simulink model "ftm_incremental_encoder_s32k1xx"  (Simulink 9.0)
settings: Solver=FixedStepDiscrete  StartTime=0.0  StopTime=10.0  FixedStep=0.01  RelTol=1e-3  EnableMultiTasking=on
model workspace (MAT data in the model file):
  FTM_Max_Counter = 4096
  Number_of_Divisions = 1024
  Sampling_Time = 0.01
  Scale_Factor : num (value not decoded)
InitFcn:
  | mbd_s32k_consistency_checks(bdroot(gcs));
undefined symbols (not defined in the file): LQFP
libraries: mbd_s32k1xx_ec_toolbox x7, simulink x1
Description:
  | This model shows FlexTimer's Quadrature Decoder Mode.
  | 
  | The Quadrature Encoder signals of a running motor are emulated using the
  | block called "Signal_Generation" using the FTM PWM. The FTM PWM writes
  | the output on the pins PTD15, and PTD0.
  | 
  | The FTM Quadrature Decoder block has as input the pins PTA1, and PTB2.
  | 
  | For the example to work connect PTA1 to PTD15 and PTB2 to PTD0.
  | 
  | This example has also a FreeMaster project associated, which is called
  | "ftm_incremental_encoder_s32k1xx.pmp".
  | 
  | For a given value of "Speed_Command" variable the pins PTD15, and PTD0
  | will be the same values as the signals of Quadrature Encoder of a
  | spinning motor at the speed "Speed_Command". It's value can be modified
  | from FreeMaster.
  | 
  | Validation: In FreeMaster "Motor_Speed" should be equal to "Speed_Command".
settings Model: Creator=NXP MBDT Team  LastModifiedBy=nxf35172  OrderedModelArguments=off
settings DataIOCC: ExternalInput=off  InitialState=off  LimitDataPoints=on  SaveOutput=off  SignalLogging=off  SaveTime=off
settings OptimizationCC: DefaultParameterBehavior=Inlined  LifeSpan=1
settings DebuggingCC: SolverPrmCheckMsg=warning  InheritedTsInSrcMsg=none  SingleTaskRateTransMsg=error  UnconnectedInputMsg=error  UnconnectedOutputMsg=error  UnconnectedLineMsg=error  AllowSymbolicDim=off  UnknownTsInhSupMsg=error  StateNameClashWarn=warning
settings HardwareCC: ProdLargestAtomicInteger=Long  ProdLargestAtomicFloat=Double  ProdEndianess=LittleEndian  ProdHWDeviceType=ARM Compatible->ARM Cortex
settings SFSimCC: MATLABDynamicMemAlloc=off
settings RTWCC: SystemTargetFile=mbd_s32k.tlc  MakeCommand=mbd_s32k_make_rtw COPY_MDLREF_INCLUDES=0  TemplateMakefile=mbd_s32k.tmf  Description=Model Based Design Toolbox S32K14x Code Generation Target  GenerateReport=on  LaunchReport=on
settings CodeAppCC: IgnoreCustomStorageClasses=off
settings STFCustomTargetCC: CombineOutputUpdateFcns=on  ERTCustomFileBanners=on  SupportContinuousTime=off  SupportNonInlinedSFcns=off  RemoveResetFunc=on  MATLABClassNameForMDSCustomization=Simulink.SoftwareTarget.ERTCustomization  GRTInterface=off  SystemTargetFile=mbd_s32k14.tlc
settings ERTTargetCC: MultiwordLength=2048  ParMdlRefBuildCompliant=off  CompOptLevelCompliant=off  ConcurrentExecutionCompliant=off  ModelStepFunctionPrototypeControlCompliant=off  CPPClassGenCompliant=off  UseToolchainInfoCompliant=off  InlinedParameterPlacement=NonHierarchical  ERTCustomFileTemplate=example_file_process.tlc  ConvertIfToSwitch=off  SuppressUnreachableDefaultCases=off

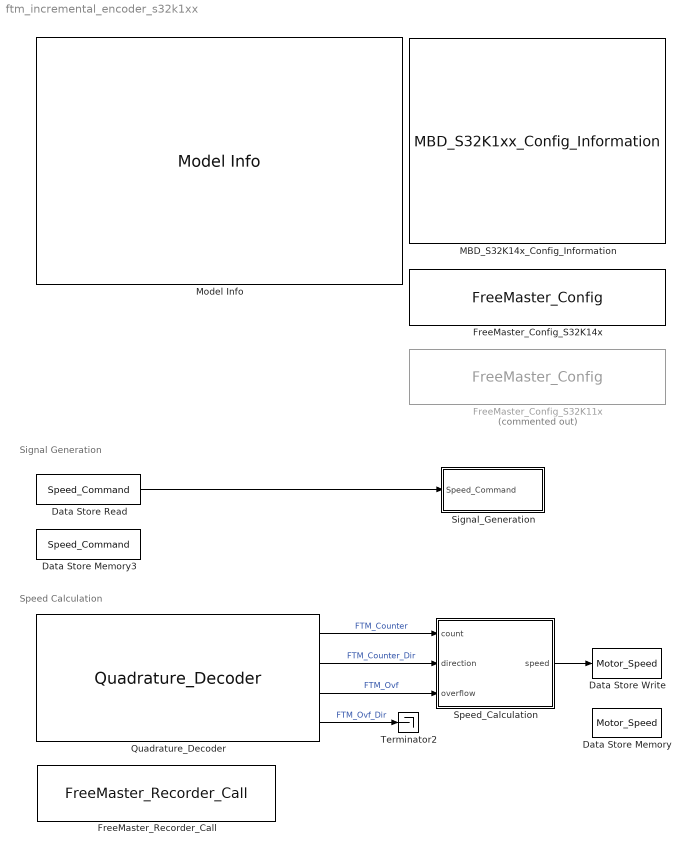
== system ftm_incremental_encoder_s32k1xx ==
  note: Signal Generation
  note: Speed Calculation
  Data Store Memory : DataStoreMemory  DataStoreName=Motor_Speed  ReadBeforeWriteMsg=warning  WriteAfterWriteMsg=warning  WriteAfterReadMsg=warning  ShowAdditionalParam=off
  Data Store Memory3 : DataStoreMemory  DataStoreName=Speed_Command  ReadBeforeWriteMsg=warning  WriteAfterWriteMsg=warning  WriteAfterReadMsg=warning  InitialValue=500  ShowAdditionalParam=off  OutDataTypeStr=single
  Data Store Read : DataStoreRead  DataStoreName=Speed_Command
  Data Store Write : DataStoreWrite  DataStoreName=Motor_Speed  DataStoreElements=Motor_Speed
  FreeMaster_Config_S32K11x : mbd_s32k1xx_ec_toolbox/Utility Blocks/FreeMaster_Config  Commented=on  interface=LPUART0  baudrate=57600  rxd=PTB0: [LPUART0_RX | Receive]  txd=PTB1: [LPUART0_TX | Transmit]  mode=Short Interrupt  isr_prio=1  show_adv_opts=on  use_scope=on  max_scope_vars=8  use_recorder=on  max_rec_vars=8  rec_buff_size=1024  rec_timebase=0 milliseconds  comm_buffer_size_auto=on  comm_buffer_size=255  comm_rqueue_size_default=on  comm_rqueue_size=32
  FreeMaster_Config_S32K14x : mbd_s32k1xx_ec_toolbox/Utility Blocks/FreeMaster_Config  interface=LPUART1  baudrate=57600  rxd=PTC6: [LPUART1_RX | Receive]  txd=PTC7: [LPUART1_TX | Transmit]  mode=Short Interrupt  isr_prio=1  show_adv_opts=on  use_scope=on  max_scope_vars=8  use_recorder=on  max_rec_vars=8  rec_buff_size=1024  rec_timebase=0 milliseconds  comm_buffer_size_auto=on  comm_buffer_size=255  comm_rqueue_size_default=on  comm_rqueue_size=32
  FreeMaster_Recorder_Call : mbd_s32k1xx_ec_toolbox/Utility Blocks/FreeMaster_Recorder_Call
  MBD_S32K14x_Config_Information : mbd_s32k1xx_ec_toolbox/MBD_S32K1xx_Config_Information  mbdt_ver=0  disp_str=|  config_params=[]  mcu_target_name=S32K146  mcu_target_package=144-LQFP  mcu_target_sram_size=128KB  mcu_system_clock_freq=80  mcu_xtal_freq=External 8  mcu_steptick_timer=LPIT Channel 0  mcu_steptick_prio=0  ds_import_enable=on  target_compiler=GCC  target_memory=FLASH  gcc_target_compile_opts=-mcpu=cortex-m4 -mthumb -mfloat-abi=hard -mfpu=fpv4-sp-d16 -O1 -g -gstrict-dwarf  gcc_target_assemble_opts=-mcpu=cortex-m4 -mthumb -mfloat-abi=hard -mfpu=fpv4-sp-d16 -g  gcc_target_link_opts=-mcpu=cortex-m4 -mthumb -mfloat-abi=hard -mfpu=fpv4-sp-d16  gcc_target_default_lcf=on  gcc_target_user_lcf=S32K146_128_flash.ld  ghs_target_compile_opts=-cpu=cortexm4f -thumb -DARM_MATH_CM4 -fpu=vfpv4_d16 -fsingle -Ogeneral -Wundef -Wimplicit-int -Wshadow -Wtrigraphs --no_commons --gnu_asm -gnu99 -gdwarf-2 -G  ghs_target_assemble_opts=-cpu=cortexm4f -fpu=vfpv4_d16  ghs_target_link_opts=-cpu=cortexm4f -thumb -fpu=vfpv4_d16  ghs_target_default_lcf=off  ghs_target_user_lcf=S32K146_128_flash.ld  iar_target_compile_opts=--cpu=Cortex-M4F --thumb --fpu=VFPv4_sp -Ol -e --debug --dlib_config normal  iar_target_assemble_opts=--cpu Cortex-M4F --thumb --fpu VFPv4_sp  iar_target_link_opts=--no_exceptions --vfe --inline  iar_target_default_lcf=off  iar_target_user_lcf=S32K146_128_flash.icf  pil_download_enable=off  rbl_download_enable=on  rbl_start_delay=5000000  rbl_download_interface=OpenSDA  rbl_restart_request=off  rbl_com_port=Custom  rbl_com_port_custom=COM1  pil_download_rate=57600  pil_opensda_drive=Custom  pil_opensda_drive_custom=D  pil_uart_instance=0  pil_uart_rx=PTA2: [LPUART0_RX | Receive]  pil_uart_tx=PTA3: [LPUART0_TX | Transmit]  FTM_PWM_PcrCheckEnDis=on  FTM_Input_Edge_Inputs_PcrCheckEnDis=on  FTM_Dual_Edge_Inputs_PcrCheckEnDis=on  FTM_Quadrature_Inputs_PcrCheckEnDis=on  FTM_Hall_Sensor_Inputs_PcrCheckEnDis=on  LPTMR_PcrCheckEnDis=on  PIT_PcrCheckEnDis=on  RTC_PcrCheckEnDis=on  FlexCAN_PcrCheckEnDis=on  LIN_PcrCheckEnDis=on  FlexIO_PcrCheckEnDis=on  LPI2C_PcrCheckEnDis=on  LPSPI_PcrCheckEnDis=on  LPUART_PcrCheckEnDis=on  CMP_PcrCheckEnDis=on  GPIO_OutputPcrCheckEnDis=on  GPIO_InputPcrCheckEnDis=on  SBC_PcrCheckEnDis=on  AMMCLIB_PcrCheckEnDis=on  FM_PcrCheckEnDis=on  Profile_PcrCheckEnDis=on  ConfigParams_PcrCheckEnDis=on  ModelRef_PcrCheckEnDis=on  PDB0_PcrCheckEnDis=on  CSEc_PcrCheckEnDis=on  eDMA_PcrCheckEnDis=on  ADC_PcrCheckEnDis=on  WDOG_PcrCheckEnDis=on
      | Target : S32K144-48KB_SRAM
      | Package : 100-pin
      | System clock : 80 MHz
      | XTAL clock : External 8 MHz
      | Compiler : IAR
      | Target Type : FLASH
      | Download Code after build : off
      | Step Tick Interrupt Priority : 15
  Model Info : simulink/Model-Wide Utilities/Model Info  Frame=off  DisplayStringWithTags=|  HorizontalTextAlignment=Left  LeftAlignmentValue=0.02
      | Model Name: %<ModelName>
      | 
      | Description: %<Description>
  Quadrature_Decoder : mbd_s32k1xx_ec_toolbox/Motor Control Blocks/FTM Blocks/Quadrature_Decoder  Priority=1  ftmModule=1  ec_mode=Phase A and Phase B  prescaler=1  cntin=0  mod=4096  phA_filtr_en=off  phA_filter=0  phA_pin=PTA1: [FTM1_QD_PHA | FTM quadrature Decode PhaseA]  polA=Normal  phB_filtr_en=off  phB_filter=0  phB_pin=PTB2: [FTM1_QD_PHB | FTM quadrature Decode PhaseB]  polB=Normal
  Signal_Generation : Subsystem
  Speed_Calculation : Subsystem
  Terminator2 : Terminator
  wires:
  Quadrature_Decoder/1 -> Speed_Calculation/1(count)  "FTM_Counter"
  Quadrature_Decoder/2 -> Speed_Calculation/2(direction)  "FTM_Counter_Dir"
  Quadrature_Decoder/3 -> Speed_Calculation/3(overflow)  "FTM_Ovf"
  Quadrature_Decoder/4 -> Terminator2/1  "FTM_Ovf_Dir"
  Speed_Calculation/1(speed) -> Data Store Write/1
  Data Store Read/1 -> Signal_Generation/1(Speed_Command)

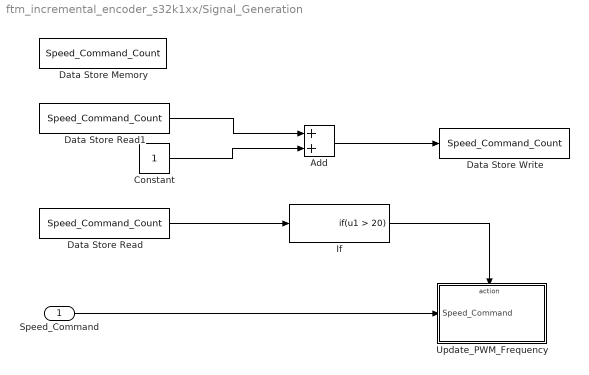
== system ftm_incremental_encoder_s32k1xx/Signal_Generation ==
  Speed_Command : Inport
  Add : Sum
  Constant : Constant
  Data Store Memory : DataStoreMemory  DataStoreName=Speed_Command_Count  ReadBeforeWriteMsg=warning  WriteAfterWriteMsg=warning  WriteAfterReadMsg=warning  ShowAdditionalParam=off
  Data Store Read : DataStoreRead  Priority=0  DataStoreName=Speed_Command_Count  DataStoreElements=Speed_Command_Count
  Data Store Read1 : DataStoreRead  DataStoreName=Speed_Command_Count  DataStoreElements=Speed_Command_Count
  Data Store Write : DataStoreWrite  DataStoreName=Speed_Command_Count  DataStoreElements=Speed_Command_Count
  If : If  IfExpression=u1 > 20  ShowElse=off
  Update_PWM_Frequency : Subsystem  TreatAsAtomicUnit=on
  wires:
  Speed_Command/1 -> Update_PWM_Frequency/1(Speed_Command)
  If/1 -> Update_PWM_Frequency/Action
  Data Store Read/1 -> If/1
  Data Store Read1/1 -> Add/1
  Constant/1 -> Add/2
  Add/1 -> Data Store Write/1

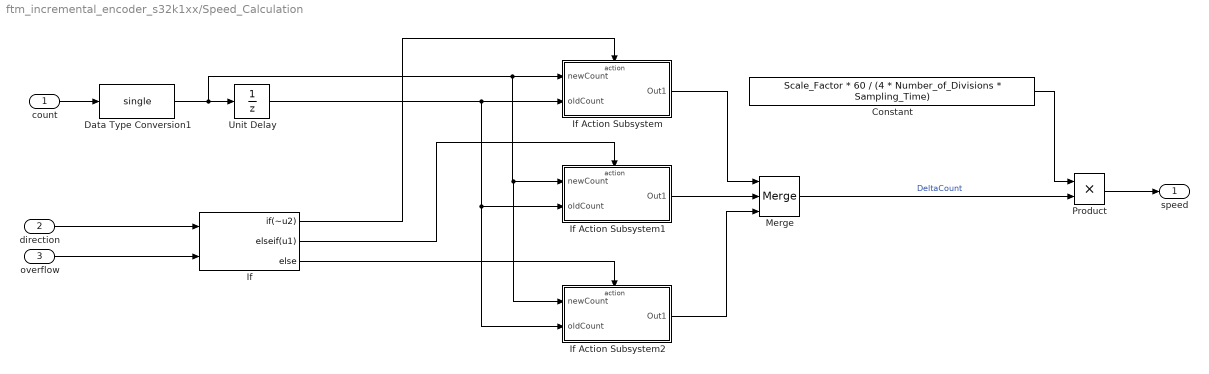
== system ftm_incremental_encoder_s32k1xx/Speed_Calculation ==
  count : Inport
  direction : Inport  Port=2
  overflow : Inport  Port=3
  Constant : Constant  Value=Scale_Factor * 60 / (4 * Number_of_Divisions * Sampling_Time)  OutDataTypeStr=single
  Data Type Conversion1 : DataTypeConversion  OutDataTypeStr=single
  If : If  NumInputs=2  IfExpression=~u2  ElseIfExpressions=u1
  If Action Subsystem : Subsystem  TreatAsAtomicUnit=on
  If Action Subsystem1 : Subsystem  TreatAsAtomicUnit=on
  If Action Subsystem2 : Subsystem  TreatAsAtomicUnit=on
  Merge : Merge  Inputs=3
  Product : Product  OutDataTypeStr=single
  Unit Delay : UnitDelay  SampleTime=-1
  speed : Outport
  wires:
  Constant/1 -> Product/1
  Product/1 -> speed/1
  count/1 -> Data Type Conversion1/1
  Data Type Conversion1/1 -> If Action Subsystem2/1(newCount), If Action Subsystem1/1(newCount), If Action Subsystem/1(newCount), Unit Delay/1
  direction/1 -> If/1
  overflow/1 -> If/2
  If/1 -> If Action Subsystem/Action
  If/2 -> If Action Subsystem1/Action
  If/3 -> If Action Subsystem2/Action
  Unit Delay/1 -> If Action Subsystem2/2(oldCount), If Action Subsystem1/2(oldCount), If Action Subsystem/2(oldCount)
  If Action Subsystem/1(Out1) -> Merge/1
  If Action Subsystem1/1(Out1) -> Merge/2
  If Action Subsystem2/1(Out1) -> Merge/3
  Merge/1 -> Product/2  "DeltaCount"

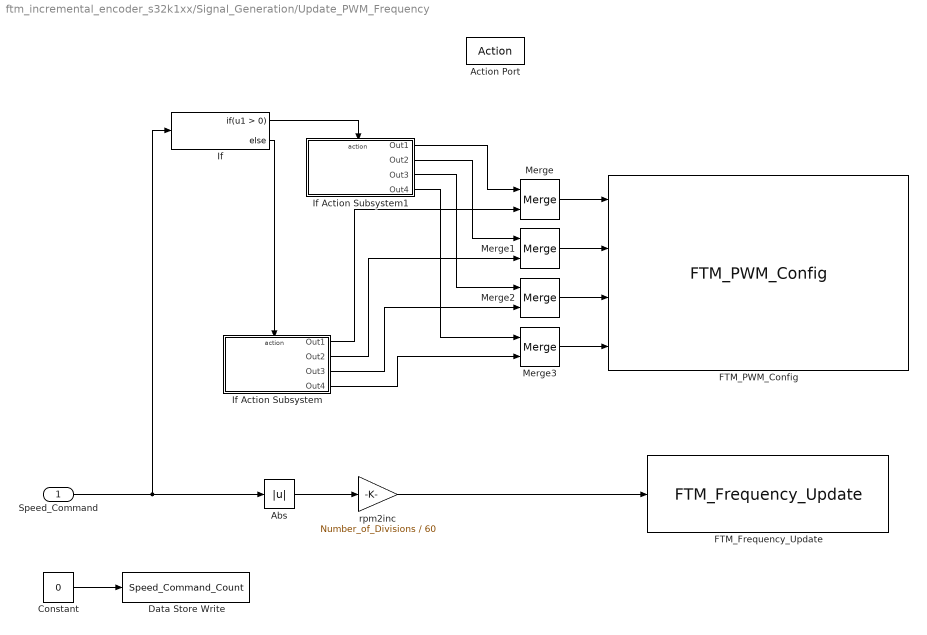
== system ftm_incremental_encoder_s32k1xx/Signal_Generation/Update_PWM_Frequency ==
  Speed_Command : Inport
  Action Port : ActionPort
  Abs : Abs
  Constant : Constant  Value=0
  Data Store Write : DataStoreWrite  DataStoreName=Speed_Command_Count  DataStoreElements=Speed_Command_Count
  FTM_Frequency_Update : mbd_s32k1xx_ec_toolbox/Motor Control Blocks/FTM Blocks/FTM_Frequency_Update  Priority=1  ftmModule=0  mcuTargetUpdate=on  ftmPwmUnits=Hz
  FTM_PWM_Config : mbd_s32k1xx_ec_toolbox/Motor Control Blocks/FTM Blocks/FTM_PWM_Config  ftmModule=0  ftmMode=Combine mode PWM  ftmSourceClock=80 MHz  swcontrol_enable=off  chan0En=on  chan0Type=Independent  chan2En=on  chan2Type=Independent  chan4En=off  chan4Type=Independent  chan6En=off  chan6Type=Independent  ftmPwmUnits=Hz  outFrequency=5000  ftmPeriod=16000  ftmPrescaler=Divide by 1  deadtimeUnits=Nanoseconds  deadtimeNs=0  deadtimeTicks=0  deadtimePrescaler=Divide by 1  dutyCycleCh0=0.5  dutyCycleCh1=0.99  dutyCycleCh2=0.25  dutyCycleCh3=0.75  dutyCycleCh4=0.25  dutyCycleCh5=0.25  dutyCycleCh6=0.25  dutyCycleCh7=0.25  dutyCycleSim=off  startAfterInit=on  showAdvOpt=on  pinFtmCh0=PTD15: [FTM0_CH0 | FTM Channel]  pinFtmCh1=None  pinPolCh0=Active High  pinPolCh1=Active Low  outputComplem0=Main duplicated  outputLevel0=Low  outputLevel1=Low  pinFtmCh2=PTD0: [FTM0_CH2 | FTM Channel]  pinFtmCh3=None  pinPolCh2=Active High  pinPolCh3=Active Low  outputComplem2=Main duplicated  outputLevel2=Low  outputLevel3=Low  pinFtmCh4=PTB4: [FTM0_CH4 | FTM Channel]  pinFtmCh5=None  pinPolCh4=Active Low  pinPolCh5=Active Low  outputComplem4=Main duplicated  outputLevel4=Low  outputLevel5=Low  pinFtmCh6=PTE8: [FTM0_CH6 | FTM Channel]  pinFtmCh7=None  pinPolCh6=Active Low  pinPolCh7=Active Low  outputComplem6=Main duplicated  outputLevel6=Low  outputLevel7=Low  initTrigger=off  chTrigger0=off  chTrigger1=off  chTrigger2=off  chTrigger3=off  chTrigger4=off  chTrigger5=off  chTrigger6=off  chTrigger7=off  mcuTargetUpdate=on  pwmSyncTrg=Software trigger  pwmSyncHwRouting=TRGMUX_FTM7  pwmSyncTrg0=off  pwmSyncTrg1=off  pwmSyncTrg2=off  pwmSyncAutoClear=on  pwmSyncMinLoad=on  pwmSyncMaxLoad=on  pwmSyncInvert=System Clock  pwmSyncOutControl=System Clock  pwmSyncOutMask=System Clock  pwmSyncCounterInitial=System Clock  pwmSyncPoints=Update now  reloadEnable=off  reloadPriority=0  reloadHalfCycle=off  reloadHCR=0  reloadFrequency=0  chnMatch0=off  chnMatch1=off  chnMatch2=off  chnMatch3=off  chnMatch4=off  chnMatch5=off  chnMatch6=off  chnMatch7=off  pwmFaultProtection=off  pwmFaultInterrupt=off  pwmFaultClearing=Fault control disabled  pwmFaultPinState=Safe Value  pwmFaultFilterValue=0  pwmFaultPriority=0  fault_disen_0=off  fault_filter_0=off  fault_polarity_0=Active High  fault_disen_1=off  fault_filter_1=off  fault_polarity_1=Active high  fault_disen_2=off  fault_filter_2=off  fault_polarity_2=Active high  fault_disen_3=off  fault_filter_3=off  fault_polarity_3=Active high  fault_pin_0=None  fault_pin_1=None  fault_pin_2=None  fault_pin_3=None
  If : If
  If Action Subsystem : Subsystem  TreatAsAtomicUnit=on
  If Action Subsystem1 : Subsystem  TreatAsAtomicUnit=on
  Merge{,1..3} (4 alike) : Merge
  rpm2inc : Gain  Gain=Number_of_Divisions / 60  OutDataTypeStr=uint32
  wires:
  Constant/1 -> Data Store Write/1
  If Action Subsystem/2(Out2) -> Merge1/2
  If Action Subsystem/4(Out4) -> Merge3/2
  If Action Subsystem1/3(Out3) -> Merge2/1
  Merge2/1 -> FTM_PWM_Config/3
  Merge3/1 -> FTM_PWM_Config/4
  If Action Subsystem/3(Out3) -> Merge2/2
  Merge1/1 -> FTM_PWM_Config/2
  Speed_Command/1 -> Abs/1, If/1
  Abs/1 -> rpm2inc/1
  If/1 -> If Action Subsystem1/Action
  If/2 -> If Action Subsystem/Action
  If Action Subsystem1/1(Out1) -> Merge/1
  Merge/1 -> FTM_PWM_Config/1
  If Action Subsystem1/2(Out2) -> Merge1/1
  If Action Subsystem/1(Out1) -> Merge/2
  rpm2inc/1 -> FTM_Frequency_Update/1
  If Action Subsystem1/4(Out4) -> Merge3/1

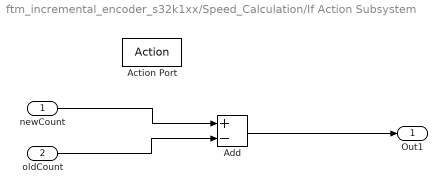
== system ftm_incremental_encoder_s32k1xx/Speed_Calculation/If Action Subsystem ==
  newCount : Inport
  oldCount : Inport  Port=2
  Action Port : ActionPort
  Add : Sum  Inputs=+-
  Out1 : Outport
  wires:
  oldCount/1 -> Add/2
  newCount/1 -> Add/1
  Add/1 -> Out1/1

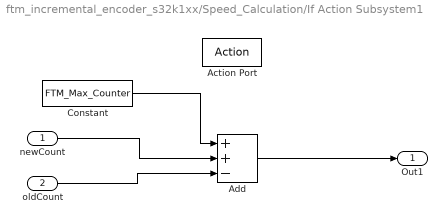
== system ftm_incremental_encoder_s32k1xx/Speed_Calculation/If Action Subsystem1 ==
  newCount : Inport
  oldCount : Inport  Port=2
  Action Port : ActionPort
  Add : Sum  Inputs=++-
  Constant : Constant  Value=FTM_Max_Counter  OutDataTypeStr=single
  Out1 : Outport
  wires:
  oldCount/1 -> Add/3
  newCount/1 -> Add/2
  Add/1 -> Out1/1
  Constant/1 -> Add/1

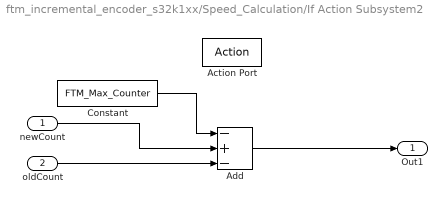
== system ftm_incremental_encoder_s32k1xx/Speed_Calculation/If Action Subsystem2 ==
  newCount : Inport
  oldCount : Inport  Port=2
  Action Port : ActionPort
  Add : Sum  Inputs=-+-
  Constant : Constant  Value=FTM_Max_Counter  OutDataTypeStr=single
  Out1 : Outport
  wires:
  oldCount/1 -> Add/3
  newCount/1 -> Add/2
  Add/1 -> Out1/1
  Constant/1 -> Add/1

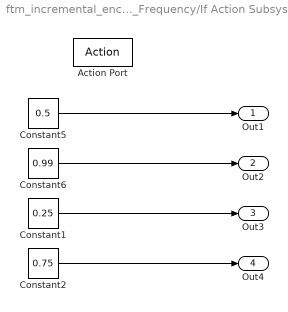
== system ftm_incremental_encoder_s32k1xx/Signal_Generation/Update_PWM_Frequency/If Action Subsystem ==
  Action Port : ActionPort
  Constant1 : Constant  Value=0.25  OutDataTypeStr=single
  Constant2 : Constant  Value=0.75  OutDataTypeStr=single
  Constant5 : Constant  Value=0.5  OutDataTypeStr=single
  Constant6 : Constant  Value=0.99  OutDataTypeStr=single
  Out1 : Outport
  Out2 : Outport  Port=2
  Out3 : Outport  Port=3
  Out4 : Outport  Port=4
  wires:
  Constant6/1 -> Out2/1
  Constant5/1 -> Out1/1
  Constant2/1 -> Out4/1
  Constant1/1 -> Out3/1

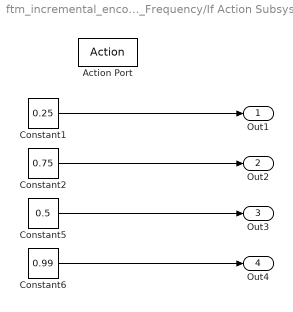
== system ftm_incremental_encoder_s32k1xx/Signal_Generation/Update_PWM_Frequency/If Action Subsystem1 ==
  Action Port : ActionPort
  Constant1 : Constant  Value=0.25  OutDataTypeStr=single
  Constant2 : Constant  Value=0.75  OutDataTypeStr=single
  Constant5 : Constant  Value=0.5  OutDataTypeStr=single
  Constant6 : Constant  Value=0.99  OutDataTypeStr=single
  Out1 : Outport
  Out2 : Outport  Port=2
  Out3 : Outport  Port=3
  Out4 : Outport  Port=4
  wires:
  Constant1/1 -> Out1/1
  Constant2/1 -> Out2/1
  Constant5/1 -> Out3/1
  Constant6/1 -> Out4/1
